simulink model "RealTime_UDP_Receive"  (R2013b)
settings: Solver=ode5  StartTime=0.0  StopTime=inf  FixedStep=0.005  RelTol=1e-3
undefined symbols (not defined in the file): Standard_Devices, UDP_Protocol
libraries: rtwinlib x1, simulink x1
settings Model: xpc_rtwmakecfg_data=_xpciplib__xpcnblib__xpcetherlib__xpcether8255xlib__xpcetherGbElib_  SimulationMode=external  ExtModeTrigDuration=120000  Creator=Mina  LastModifiedBy=Mina
settings HardwareCC: ProdIntDivRoundTo=Zero  ProdEndianess=LittleEndian  ProdHWDeviceType=Generic->32-bit x86 compatible
settings RTWCC: SystemTargetFile=rtwin.tlc  TemplateMakefile=rtwin.tmf  Description=Real-Time Windows Target  ProcessScript=rtwin_make_rtw_hook  RTWCompilerOptimization=On
settings CodeAppCC: MaxIdLength=95
settings RTWinTargetCC: TargetLibSuffix=_rtwin.lib  TargetPreCompLibLocation=F:\Program Files\MATLAB\R2013b\toolbox\rtw\targets\rtwin\lib\win64  CodeReplacementLibrary=ANSI_C  RTWinDir=F:/PROGRA~1/MATLAB/R2013b/toolbox/rtw/targets/rtwin  TargetArch=win64

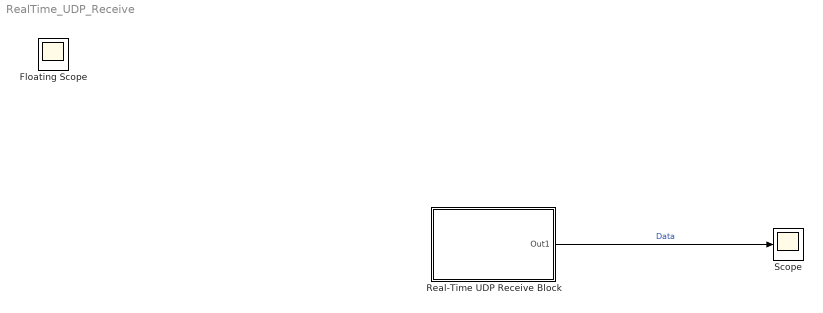
== system RealTime_UDP_Receive ==
  Real-Time UDP Receive Block : Subsystem
  Scope : Scope
      settings: TimeRange=60  YMin=-3000  YMax=3000  SaveName=ScopeData2  MaxDataPoints=500000  SampleInput=on  SampleTime=0.005
  Floating Scope : Scope
      settings: Floating=on
  wires:
  Real-Time UDP Receive Block/1(Out1) -> Scope/1  "Data"

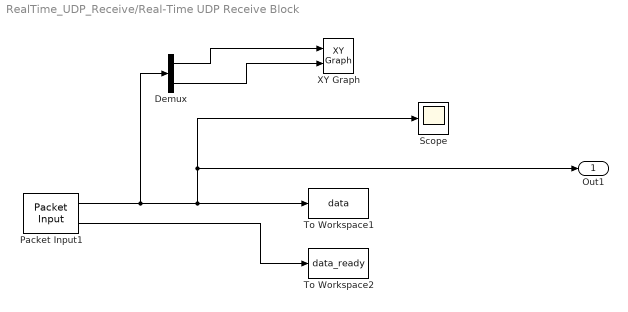
== system RealTime_UDP_Receive/Real-Time UDP Receive Block ==
  Demux : Demux  Outputs=2
  Packet Input1 : rtwinlib/Packet Input  SampleTime=0.005  MaxMissedTicks=1000  ShowMissedTicks=off  YieldWhenWaiting=off  DrvName=Standard_Devices/UDP_Protocol  DrvAddress=33433  DrvOptions=[2130706433 12000]  PacketSize=16  DataTypes='2*double'  ShowReady=on  ShowError=off  PacketID=1  ByteOrder=1  ShowTimestamp=off
      settings: AttributesFormatString=Standard Devices\nUDP Protocol [8299h]
  Scope : Scope
      settings: TimeRange=60  YMin=-3000  YMax=3000  MaxDataPoints=500000  SampleInput=on  SampleTime=0.005
  To Workspace1 : ToWorkspace  VariableName=data  SampleTime=-1  SaveFormat=Structure With Time
  To Workspace2 : ToWorkspace  VariableName=data_ready  SampleTime=-1  SaveFormat=Structure With Time
  XY Graph : simulink/Sinks/XY Graph  xmin=-3000  xmax=3000  ymin=-2000  ymax=2000  st=0.005
  Out1 : Outport
  wires:
  Packet Input1/2 -> To Workspace2/1
  Packet Input1/1 -> Demux/1, Out1/1, Scope/1, To Workspace1/1
  Demux/2 -> XY Graph/2
  Demux/1 -> XY Graph/1
